simulink model "psa_lab02"  (R2018a)
settings: Solver=VariableStepAuto  StartTime=0.0  StopTime=0.2  RelTol=1e-3
libraries: powerlib x8, powerlib_meascontrol x2
settings Model: Creator=Rehan Qasim  LastModifiedBy=Rehan Qasim

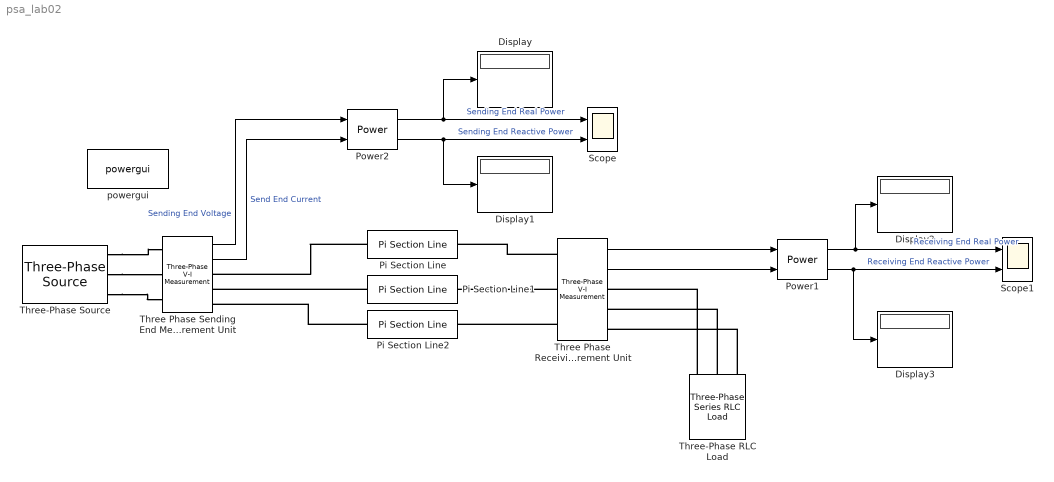
== system psa_lab02 ==
  Display{,1..3} (4 alike) : Display
  Pi Section Line : powerlib/Elements/Pi Section Line  LConnTagsString=__new0  RConnTagsString=__new0  Frequency=50  Resistance=1e-9  Inductance=2e-3  Capacitance=8e-9  Length=400  PiSections=1  Measurements=None
      settings: AttributesFormatString=\n  SourceProductName=Simscape Power Systems  SourceProductBaseCode=PS
  Pi Section Line1 : powerlib/Elements/Pi Section Line  LConnTagsString=__new0  RConnTagsString=__new0  Frequency=50  Resistance=1e-8  Inductance=2e-3  Capacitance=8e-9  Length=400  PiSections=1  Measurements=None
      settings: AttributesFormatString=\n  SourceProductName=Simscape Power Systems  SourceProductBaseCode=PS
  Pi Section Line2 : powerlib/Elements/Pi Section Line  LConnTagsString=__new0  RConnTagsString=__new0  Frequency=50  Resistance=1e-9  Inductance=2e-3  Capacitance=8e-9  Length=400  PiSections=1  Measurements=None
      settings: AttributesFormatString=\n  SourceProductName=Simscape Power Systems  SourceProductBaseCode=PS
  Power1 : powerlib_meascontrol/Measurements/Power  Freq=50  Vinit=[1, 0]  Iinit=[1, 0]  Ts=0
      settings: SourceProductName=Simscape Power Systems
  Power2 : powerlib_meascontrol/Measurements/Power  Freq=50  Vinit=[1, 0]  Iinit=[1, 0]  Ts=0
      settings: SourceProductName=Simscape Power Systems
  Scope : Scope  NumInputPorts=2
  Scope1 : Scope  NumInputPorts=2
  "Three Phase Receiving End Measurement Unit  " : powerlib/Measurements/Three-Phase V-I Measurement  VoltageMeasurement=phase-to-ground  SetLabelV=off  LabelV=Vabc  Vpu=off  VpuLL=off  CurrentMeasurement=yes  SetLabelI=off  LabelI=Iabc  Ipu=off  Pbase=100e6  Vbase=500e3  OutputType=Complex  PhasorSimulation=off  PSBequivalent=0
  "Three Phase Sending End Measurement Unit  " : powerlib/Measurements/Three-Phase V-I Measurement  VoltageMeasurement=phase-to-ground  SetLabelV=off  LabelV=Vabc  Vpu=off  VpuLL=off  CurrentMeasurement=yes  SetLabelI=off  LabelI=Iabc  Ipu=off  Pbase=100e6  Vbase=500e3  OutputType=Complex  PhasorSimulation=off  PSBequivalent=0
  Three-Phase RLC Load : powerlib/Elements/Three-Phase Series RLC Load  LConnTagsString=A|B|C  Configuration=Y (grounded)  NominalVoltage=238e3  Vabc=[1e3 1e3 1e3]  Vabcp=[1e3 1e3 1e3]  NominalFrequency=50  UnbalancedPower=off  ActivePower=100.00e6  InductivePower=0  CapacitivePower=0  Pabc=[10e3 9e3 11e3]  QLabc=[100 90 110]  QCabc=[100 90 110]  Pabcp=[10e3 9e3 11e3]  QLabcp=[100 90 110]  QCabcp=[100 90 110]  Measurements=None  LoadType=constant Z
  Three-Phase Source : powerlib/Electrical Sources/Three-Phase Source  InternalConnection=Yg  VoltagePhases=off  Voltage=238e3  PhaseAngle=0  Voltage_phases=[25e3 25e3 25e3]/sqrt(3)  PhaseAngles_phases=[0 -120 +120]  Frequency=50  NonIdealSource=on  SpecifyImpedance=off  Resistance=.00001  Inductance=16.58e-9  ShortCircuitLevel=100e6  BaseVoltage=25e3  XRratio=7  BusType=swing  Pref=10e3  Qref=0  Prefabc=[10e3, 10e3, 10e3]  Qrefabc=[0, 0, 0]  Qmin=-inf  Qmax=inf
  powergui : powerlib/powergui  Priority=1  SimulationMode=Continuous  SampleTime=50e-6  frequency=60  Iterations=50  frequencyindice=50  Pbase=100e6  ErrMax=1e-4  UnitsV=kV  UnitsW=MW  buscounter=0  FunctionMessages=off  echomessages=off  EnableUseOfTLC=off  CurrentSourceSwitches=off  DisableSnubberDevices=off  DisableRonSwitches=off  DisableVfSwitches=off  DisplayEquations=off  SolverType=Tustin/Backward Euler (TBE)  Interpol=off  ExternalGateDelay=off  methode=off  Ts=100  x0status=blocks  SPID=on  SwTol=0  HookPort=off  RestoreLinks=warning  ResistiveCurrentMeasurement=off  Frange=[0:2:500]  Ylog=off  Xlog=on  ShowGrid=off  save=off  variable=ZData  structure=0  ZoomFFT=off  StartTime=0.0  cycles=1  DisplayStyle=1  fundamental=60  FreqAxis=off  MaxFrequency=1000  frequencyindicesteady=1  RmsSteady=2  display=off
  wires:
  Power1/2 -> Display3/1, Scope1/2  "Receiving End Reactive Power"
  "Three Phase Sending End Measurement Unit  "/2 -> Power2/2  "Send End Current"
  Power2/1 -> Display/1, Scope/1  "Sending End Real Power"
  "Three Phase Receiving End Measurement Unit  "/1 -> Power1/1
  "Three Phase Sending End Measurement Unit  "/1 -> Power2/1  "Sending End Voltage"
  Power2/2 -> Display1/1, Scope/2  "Sending End Reactive Power"
  "Three Phase Receiving End Measurement Unit  "/2 -> Power1/2
  Power1/1 -> Scope1/1, Display2/1  "Receiving End Real Power"
  connections:
  "Three Phase Receiving End Measurement Unit  "/LConn3 -- Pi Section Line2/RConn1
  Three-Phase RLC Load/LConn1 -- "Three Phase Receiving End Measurement Unit  "/RConn1
  Three-Phase Source/RConn3 -- "Three Phase Sending End Measurement Unit  "/LConn3
  Three-Phase Source/RConn1 -- "Three Phase Sending End Measurement Unit  "/LConn1
  "Three Phase Receiving End Measurement Unit  "/LConn2 -- Pi Section Line1/RConn1
  Three-Phase RLC Load/LConn2 -- "Three Phase Receiving End Measurement Unit  "/RConn2
  "Three Phase Receiving End Measurement Unit  "/LConn1 -- Pi Section Line/RConn1
  Three-Phase RLC Load/LConn3 -- "Three Phase Receiving End Measurement Unit  "/RConn3
  Pi Section Line2/LConn1 -- "Three Phase Sending End Measurement Unit  "/RConn3
  Pi Section Line/LConn1 -- "Three Phase Sending End Measurement Unit  "/RConn1
  Pi Section Line1/LConn1 -- "Three Phase Sending End Measurement Unit  "/RConn2
  Three-Phase Source/RConn2 -- "Three Phase Sending End Measurement Unit  "/LConn2
